simulink model "sim_2_4"  (R2023b)
settings: Solver=FixedStepAuto  StartTime=0.0  StopTime=100  FixedStep=Tc*Tf  RelTol=1e-3
values from neighbouring files (symbols this model uses):
  k1 = 1    [H2_5.m]
  k2 = 1    [H2_5.m]
undefined symbols (not defined in the file or in its folder): b, Tf
libraries: robotmobilelib x1
settings Model: Creator=Valentina Giannotti  LastModifiedBy=Valentina Giannotti

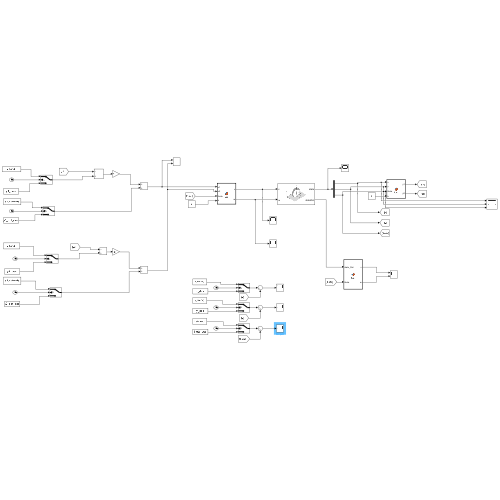
[thumbnail: Simulink's stored preview of the top-level diagram]
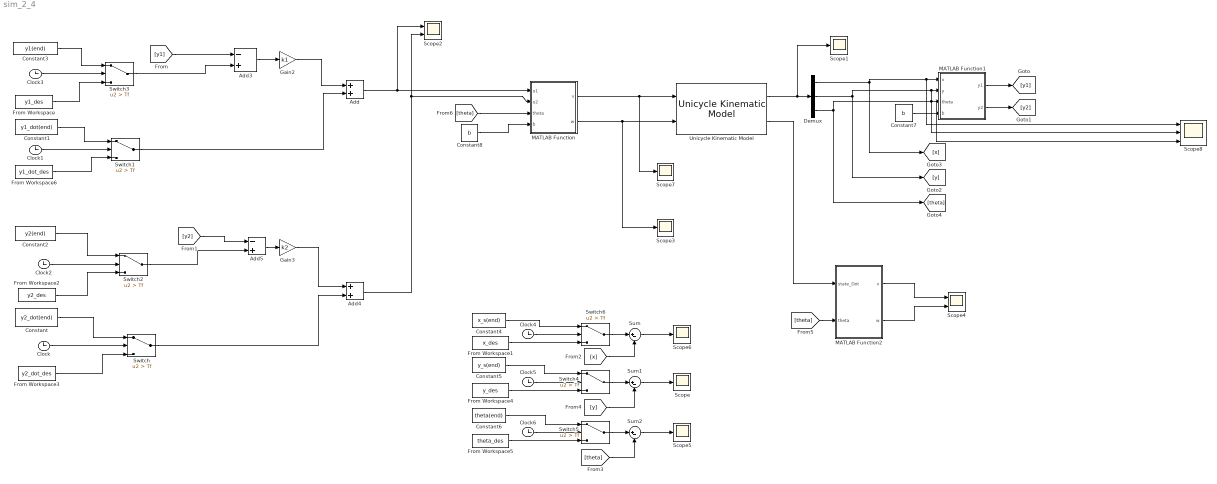
== system sim_2_4 ==
  Add : Sum
  Add3 : Sum  Inputs=-+
  Add4 : Sum
  Add5 : Sum  Inputs=-+
  Clock{,1..6} (7 alike) : Clock
  Constant : Constant  Value=y2_dot(end)
  Constant1 : Constant  Value=y1_dot(end)
  Constant2 : Constant  Value=y2(end)
  Constant3 : Constant  Value=y1(end)
  Constant4 : Constant  Value=x_s(end)
  Constant5 : Constant  Value=y_s(end)
  Constant6 : Constant  Value=theta(end)
  Constant7 : Constant  Value=b
  Constant8 : Constant  Value=b
  Demux : Demux  Outputs=3
  From Workspace : FromWorkspace  VariableName=y1_des
  From Workspace1 : FromWorkspace  VariableName=x_des
  From Workspace2 : FromWorkspace  VariableName=y2_des
  From Workspace3 : FromWorkspace  VariableName=y2_dot_des
  From Workspace4 : FromWorkspace  VariableName=y_des
  From Workspace5 : FromWorkspace  VariableName=theta_des
  From Workspace6 : FromWorkspace  VariableName=y1_dot_des
  Gain2 : Gain  Gain=k1
  Gain3 : Gain  Gain=k2
  MATLAB Function : MATLAB Function  TreatAsAtomicUnit=on
  MATLAB Function1 : MATLAB Function  TreatAsAtomicUnit=on
  MATLAB Function2 : MATLAB Function  TreatAsAtomicUnit=on
  Scope{,1,3,5..7} (6 alike) : Scope
  Scope2 : Scope  NumInputPorts=2
  Scope4 : Scope  NumInputPorts=2
  Scope8 : Scope  NumInputPorts=3
  Sum : Sum  Inputs=|+-
  Sum1 : Sum  Inputs=|+-
  Sum2 : Sum  Inputs=|+-
  Switch{,1..6} (7 alike) : Switch  Criteria=u2 > Threshold  Threshold=Tf  SaturateOnIntegerOverflow=off  InputSameDT=off
  Unicycle Kinematic Model : robotmobilelib/Unicycle Kinematic Model  VehicleInputs=Vehicle Speed & Heading Angular Velocity  WheelRadius=b  WheelSpeedRange=[-Inf Inf]  InitialState=[0; 0; 0]  SimulateUsing=Interpreted execution
  wires:
  Demux/3 -> [theta], Scope8/3, MATLAB Function1/3(theta)
  Unicycle Kinematic Model/1 -> Scope1/1, Demux/1
  Demux/2 -> [y], Scope8/2, MATLAB Function1/2(y)
  MATLAB Function/2(w) -> Scope3/1, Unicycle Kinematic Model/2
  MATLAB Function/1(v) -> Scope7/1, Unicycle Kinematic Model/1
  MATLAB Function1/1(y1) -> [y1]
  MATLAB Function1/2(y2) -> [y2]
  Add4/1 -> MATLAB Function/2(u2), Scope2/2
  From Workspace3/1 -> Switch/3
  Add5/1 -> Gain3/1
  Switch/1 -> Add4/2
  [y2] -> Add5/1
  Clock/1 -> Switch/2
  Switch2/1 -> Add5/2
  Clock2/1 -> Switch2/2
  From Workspace2/1 -> Switch2/3
  Constant/1 -> Switch/1
  Constant2/1 -> Switch2/1
  Gain3/1 -> Add4/1
  Add/1 -> MATLAB Function/1(u1), Scope2/1
  From Workspace6/1 -> Switch1/3
  From Workspace/1 -> Switch3/3
  Constant1/1 -> Switch1/1
  Add3/1 -> Gain2/1
  Clock1/1 -> Switch1/2
  Constant3/1 -> Switch3/1
  Switch1/1 -> Add/2
  Gain2/1 -> Add/1
  Clock3/1 -> Switch3/2
  Switch3/1 -> Add3/2
  [y1] -> Add3/1
  Unicycle Kinematic Model/2 -> MATLAB Function2/1(state_Dot)
  Demux/1 -> [x], Scope8/1, MATLAB Function1/1(x)
  From Workspace1/1 -> Switch6/3
  From Workspace4/1 -> Switch4/3
  From Workspace5/1 -> Switch5/3
  Clock4/1 -> Switch6/2
  Clock5/1 -> Switch4/2
  Clock6/1 -> Switch5/2
  Constant4/1 -> Switch6/1
  Constant5/1 -> Switch4/1
  Constant6/1 -> Switch5/1
  Switch6/1 -> Sum/1
  Switch5/1 -> Sum2/1
  Switch4/1 -> Sum1/1
  [y] -> Sum1/2
  [x] -> Sum/2
  [theta] -> Sum2/2
  Sum/1 -> Scope6/1
  Sum1/1 -> Scope/1
  Sum2/1 -> Scope5/1
  [theta] -> MATLAB Function2/2(theta)
  MATLAB Function2/1(v) -> Scope4/1
  MATLAB Function2/2(w) -> Scope4/2
  Constant7/1 -> MATLAB Function1/4(b)
  Constant8/1 -> MATLAB Function/4(b)
  [theta] -> MATLAB Function/3(theta)

== matlab function sim_2_4/MATLAB Function1 ==
  data: x input; y1 output; y input; theta input; y2 output; b input
function [y1 , y2] = fcn(x,y,theta,b)

y1 = x + b*cos(theta);
y2 = y + b*sin(theta);

end

== matlab function sim_2_4/MATLAB Function ==
  data: u1 input; v output; u2 input; theta input; w output; b input
function [v,w] = fcn(u1,u2,theta,b)

T=[cos(theta) -b*sin(theta); sin(theta) b*cos(theta)];
T_inv=inv(T);
f = T_inv*[u1;u2];
v=f(1);
w=f(2);
end

== matlab function sim_2_4/MATLAB Function2 ==
  data: state_Dot input; v output; w output; theta input
function [v,w] = fcn(state_Dot,theta)

w=state_Dot(3);
v=state_Dot(1)/cos(theta);

end
